simulink model "FSK"  (R2020a)
settings: Solver=VariableStepAuto  StartTime=0.0  StopTime=10.0  RelTol=1e-3
settings Model: Creator=AVS  LastModifiedBy=AVS

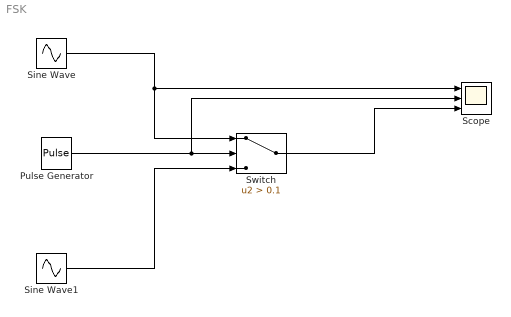
== system FSK ==
  Pulse Generator : DiscretePulseGenerator  PulseType=Time based  PulseWidth=50
  Scope : Scope  NumInputPorts=3
  Sine Wave : Sin  Frequency=50  SampleTime=0.001
  Sine Wave1 : Sin  Frequency=20  SampleTime=0.001
  Switch : Switch  Criteria=u2 > Threshold  Threshold=0.1
  wires:
  Pulse Generator/1 -> Scope/2, Switch/2
  Sine Wave1/1 -> Switch/3
  Sine Wave/1 -> Switch/1, Scope/1
  Switch/1 -> Scope/3
